simulink library "csc_est_state_est_mtv_lib"  (R2014b)
settings: Solver=ode45  StartTime=0.0  StopTime=10.0  RelTol=1e-3
values from neighbouring files (symbols this model uses):
  est_time_step = fsw_dt    [csc_kfl_kalman_filter_mtv_init.m]
libraries: simulink x1, util_info_lib x1, csc_emp_est_mass_props_lib x1, csc_kfl_kalman_filter_mtv_lib x1, csc_spc_sensor_processing_mtv_lib x1, csu_elk_est_landed_kinematics_mtv_lib x1, csu_esf_est_switch_frame_mtv_lib x1, csu_kfo_kalman_filter_output_mtv_lib x1, util_fsw_frame_rotation_lib x1
settings Model: Creator=ianmga  LastModifiedBy=mstewart

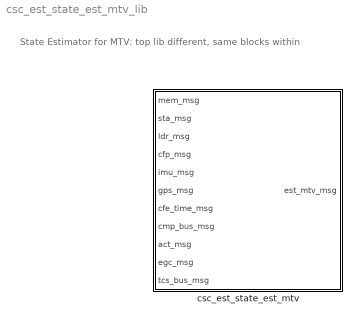
== system csc_est_state_est_mtv_lib ==
  note: State Estimator for MTV:
      | top lib different, same blocks within
  csc_est_state_est_mtv : Subsystem  Tag=OFSW; MDL_TICK=CMP_MTV_MSG  TreatAsAtomicUnit=on  SystemSampleTime=est_time_step

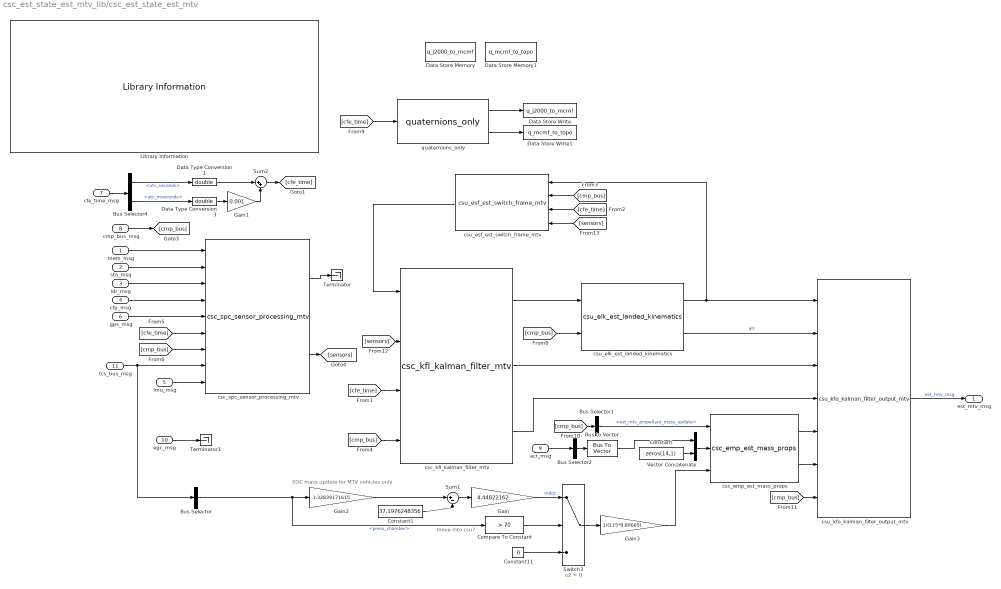
== system csc_est_state_est_mtv_lib/csc_est_state_est_mtv ==
  note: EGC mass update for MTV vehicles only
  note: move into csu?
  mem_msg : Inport  OutDataTypeStr=Bus: mem_msg
  sta_msg : Inport  Port=2  OutDataTypeStr=Bus: sta_msg
  ldr_msg : Inport  Port=3  OutDataTypeStr=Bus: ldr_msg
  cfp_msg : Inport  Port=4  OutDataTypeStr=Bus: cfp_msg
  imu_msg : Inport  Port=5  OutDataTypeStr=Bus: imu_msg
  gps_msg : Inport  Port=6  OutDataTypeStr=Bus: gps_msg
  cfe_time_msg : Inport  Port=7  OutDataTypeStr=Bus: cfe_time_msg
  cmp_bus_msg : Inport  Port=8
  act_msg : Inport  Port=9
  egc_msg : Inport  Port=10  OutDataTypeStr=Bus: egc_bus_msg
  tcs_bus_msg : Inport  Port=11  OutDataTypeStr=Bus: tcs_bus_msg
  Bus Selector : BusSelector  OutputSignals=converted_pressures.press_chamber
  Bus Selector1 : BusSelector  OutputSignals=est_mtv_propellant_mass_update
  Bus Selector2 : BusSelector  OutputSignals=coarse1_time,coarse2_time,coarse3_time,coarse4_time,coarse5_time,coarse6_time,coarse7_time,coarse8_time,coarse9_time,coarse10_time,coarse11_time,coarse12_time  OutputAsBus=on
  Bus Selector4 : BusSelector  OutputSignals=utc_seconds,utc_mseconds
  Bus to Vector : BusToVector
  Compare To Constant : simulink/Logic and Bit Operations/Compare To Constant  relop=>  const=70  OutDataTypeStr=boolean
  Constant : Constant  Value=zeros(14,1)  OutDataTypeStr=uint8
  Constant1 : Constant  Value=37.1976248356  OutDataTypeStr=double
  Constant11 : Constant  Value=0
  Data Store Memory : DataStoreMemory  DataStoreName=q_j2000_to_mcmf  ReadBeforeWriteMsg=warning  WriteAfterWriteMsg=warning  WriteAfterReadMsg=warning  InitialValue=[0 0 0 1]  OutDataTypeStr=double
  Data Store Memory1 : DataStoreMemory  DataStoreName=q_mcmf_to_topo  ReadBeforeWriteMsg=warning  WriteAfterWriteMsg=warning  WriteAfterReadMsg=warning  InitialValue=[0 0 0 1]  OutDataTypeStr=double
  Data Store Write : DataStoreWrite  DataStoreName=q_j2000_to_mcmf
  Data Store Write1 : DataStoreWrite  DataStoreName=q_mcmf_to_topo
  Data Type Conversion1 : DataTypeConversion  OutDataTypeStr=double
  Data Type Conversion3 : DataTypeConversion  OutDataTypeStr=double
  Gain : Gain  Gain=4.44822162
  Gain1 : Gain  Gain=0.001
  Gain2 : Gain  Gain=1.32839171615
  Gain3 : Gain  Gain=1/(115*9.80665)
  Library Information : util_info_lib/Library Information  owner='escrane'
  Sum1 : Sum  Inputs=|+-
  Sum2 : Sum  Inputs=|++
  Switch3 : Switch  Criteria=u2 > Threshold
  Terminator : Terminator
  Terminator1 : Terminator
  Vector Concatenate : Concatenate
  csc_emp_est_mass_props : csc_emp_est_mass_props_lib/csc_emp_est_mass_props
  csc_kfl_kalman_filter_mtv : csc_kfl_kalman_filter_mtv_lib/csc_kfl_kalman_filter_mtv
  csc_spc_sensor_processing_mtv : csc_spc_sensor_processing_mtv_lib/csc_spc_sensor_processing_mtv
  csu_elk_est_landed_kinematics : csu_elk_est_landed_kinematics_mtv_lib/csu_elk_est_landed_kinematics
  csu_esf_est_switch_frame_mtv : csu_esf_est_switch_frame_mtv_lib/csu_esf_est_switch_frame_mtv
  csu_kfo_kalman_filter_output_mtv : csu_kfo_kalman_filter_output_mtv_lib/csu_kfo_kalman_filter_output_mtv
  quaternions_only : util_fsw_frame_rotation_lib/quaternions_only  SystemSampleTime=-1
  est_mtv_msg : Outport  OutDataTypeStr=Bus: est_mtv_msg
  wires:
  egc_msg/1 -> Terminator1/1
  Compare To Constant/1 -> Switch3/2
  Constant1/1 -> Sum1/2
  Gain2/1 -> Sum1/1
  Gain/1 -> Switch3/1  "mdot"
  Constant11/1 -> Switch3/3
  Sum1/1 -> Gain/1
  Bus Selector/1 -> Compare To Constant/1, Gain2/1  "<press_chamber>"
  Switch3/1 -> Gain3/1
  imu_msg/1 -> csc_spc_sensor_processing_mtv/9
  tcs_bus_msg/1 -> csc_spc_sensor_processing_mtv/8, Bus Selector/1
  csc_kfl_kalman_filter_mtv/3 -> csu_kfo_kalman_filter_output_mtv/4
  gps_msg/1 -> csc_spc_sensor_processing_mtv/5
  [sensors] -> csc_kfl_kalman_filter_mtv/2
  csc_spc_sensor_processing_mtv/2 -> [sensors]
  [cmp_bus] -> csu_kfo_kalman_filter_output_mtv/7
  Constant/1 -> Vector Concatenate/2
  Vector Concatenate/1 -> csc_emp_est_mass_props/2
  Bus to Vector/1 -> Vector Concatenate/1
  Bus Selector2/1 -> Bus to Vector/1
  act_msg/1 -> Bus Selector2/1
  Bus Selector1/1 -> csc_emp_est_mass_props/1  "<est_mtv_propellant_mass_update>"
  [cmp_bus] -> Bus Selector1/1
  mem_msg/1 -> csc_spc_sensor_processing_mtv/1
  quaternions_only/2 -> Data Store Write1/1
  quaternions_only/1 -> Data Store Write/1
  [cfe_time] -> quaternions_only/1
  csc_spc_sensor_processing_mtv/1 -> Terminator/1
  csc_kfl_kalman_filter_mtv/2 -> csu_kfo_kalman_filter_output_mtv/3
  csu_elk_est_landed_kinematics/2 -> csu_kfo_kalman_filter_output_mtv/2  "alt"
  [sensors] -> csu_esf_est_switch_frame_mtv/4
  [cmp_bus] -> csu_elk_est_landed_kinematics/2
  csu_elk_est_landed_kinematics/1 -> csu_esf_est_switch_frame_mtv/1, csu_kfo_kalman_filter_output_mtv/1
  csc_kfl_kalman_filter_mtv/1 -> csu_elk_est_landed_kinematics/1
  [cmp_bus] -> csc_spc_sensor_processing_mtv/7
  [cmp_bus] -> csc_kfl_kalman_filter_mtv/4
  [cfe_time] -> csc_kfl_kalman_filter_mtv/3
  [cmp_bus] -> csu_esf_est_switch_frame_mtv/2
  [cfe_time] -> csu_esf_est_switch_frame_mtv/3
  cmp_bus_msg/1 -> [cmp_bus]
  csu_esf_est_switch_frame_mtv/1 -> csc_kfl_kalman_filter_mtv/1
  csu_kfo_kalman_filter_output_mtv/1 -> est_mtv_msg/1  "est_mtv_msg"
  csc_emp_est_mass_props/1 -> csu_kfo_kalman_filter_output_mtv/5
  csc_emp_est_mass_props/2 -> csu_kfo_kalman_filter_output_mtv/6
  Gain3/1 -> csc_emp_est_mass_props/3
  sta_msg/1 -> csc_spc_sensor_processing_mtv/2
  ldr_msg/1 -> csc_spc_sensor_processing_mtv/3
  cfp_msg/1 -> csc_spc_sensor_processing_mtv/4
  [cfe_time] -> csc_spc_sensor_processing_mtv/6
  Gain1/1 -> Sum2/2
  Data Type Conversion3/1 -> Gain1/1
  Data Type Conversion1/1 -> Sum2/1
  Bus Selector4/1 -> Data Type Conversion1/1  "<utc_seconds>"
  Bus Selector4/2 -> Data Type Conversion3/1  "<utc_mseconds>"
  cfe_time_msg/1 -> Bus Selector4/1
  Sum2/1 -> [cfe_time]
